simulink model "r2bb2xpfb14mcr25"  (R2012b)
settings: Solver=VariableStepDiscrete  SolverMode=SingleTasking  StartTime=0.0  StopTime=10.0  RelTol=1e-3
undefined symbols (not defined in the file): bit_reverse, pfb_coeff_gen_calc
libraries: xbsIndex_r4 x8058, casper_library_misc x54, casper_library_delays x18, xps_library x7
(part 92 of 105)

== system r2bb2xpfb14mcr25/fft_biplex_2by2_real/fft_biplex_real_2x2/biplex_core/fft_stage_14/butterfly_direct/twiddle/coeff_gen/cosin ==
  theta : Inport
  misci : Inport  Port=2
  Constant4 : xbsIndex_r4/Constant  const=0  gui_display_data_type=Fixed-point  arith_type=Unsigned  n_bits=1  bin_pt=0  preci_type=Single  exp_width=8  frac_width=24  explicit_period=on  period=1  equ=P=C  opselect=C  inp2=PCIN>>17  opr=+  inp1=P  carry=CIN  dbl_ovrd=off  block_type=constant
  Constant5 : xbsIndex_r4/Constant  const=0  gui_display_data_type=Fixed-point  arith_type=Unsigned  n_bits=1  bin_pt=0  preci_type=Single  exp_width=8  frac_width=24  explicit_period=on  period=1  equ=P=C  opselect=C  inp2=PCIN>>17  opr=+  inp1=P  carry=CIN  dbl_ovrd=off  block_type=constant
  Delay : xbsIndex_r4/Delay  rst=off  infoeditControl=Selection of Reset will increase slice count due to use of real FFs and instead of SRLs  en=off  latency=bram_latency  dbl_ovrd=off  reg_retiming=on  block_type=delay
  Delay10 : xbsIndex_r4/Delay  rst=off  infoeditControl=Selection of Reset will increase slice count due to use of real FFs and instead of SRLs  en=off  latency=bram_latency  dbl_ovrd=off  reg_retiming=on  block_type=delay
  Delay8 : xbsIndex_r4/Delay  rst=off  infoeditControl=Selection of Reset will increase slice count due to use of real FFs and instead of SRLs  en=off  latency=bram_latency  dbl_ovrd=off  reg_retiming=on  block_type=delay
  ROM : xbsIndex_r4/ROM  depth=2^(13)  initVector=[34359476224 34359738318 34359738267 34359738217 34359738167 34359738117 34359738066 34359738016 34359737966 34359737916 34359737865 34359737815 34359737765 34359475571 34359475520 34359475470 34359475420 34359213225 34359213175 34359213125 34358950931 34358950880 34358688686 34358688636 34358426442 34358426391 34358164197 34358164147 34357901953 34357901902 34357639708 34357639658 34357377464 34357377413 34357115219 34356853025 34356852975 34356590780 34356328586 34356066392 34356066341 34355804147 34355541953 34355279759 34355017564 34354755370 34354755320 34354493126 34354230931 34353968737 34353706543 34353444349 34353182154 34352919960 34352657766 34352395572 34352133377 34351871183 34351608989 34351084651 34350822456 34350560262 34350298068 34350035874 34349773679 34349249341 34348987147 34348724953 34348200614 34347938420 34347676226 34347151888 34346889693 34346627499 34346103161 34345840967 34345316628 34345054434 34344530096 34344267902 34343743563 34343481369 34342957031 34342694837 34342170498 34341646160 34341383966 34340859628 34340335289 34340073095 34339548757 34339024419 34338500081 34338237886 34337713548 34337189210 34336664872 34336140533 34335616195 34335354001 34334829663 34334305324 34333780986 34333256648 34332732310 34332207972 34331683633 34331159295 34330634957 34330110619 34329324136 34328799798 34328275460 34327751122 34327226784 34326702445 34325915963 34325391625 34324867287 34324342948 34323556466 34323032128 34322507790 34321721308 34321196969 34320410487 34319886149 34319361811 34318575329 34318050990 34317264508 34316740170 34315953688 34315429350 34314642867 34313856385 34313332047 34312545565 34311759083 34311234744 34310448262 34309661780 34309137442 34308350960 34307564477 34306777995 34306253657 34305467175 34304680693 34303894211 34303107728 34302321246 34301534764 34300748282 34299961800 34299437461 34298650979 34297602353 34296815871 34296029389 34295242907 34294456424 34293669942 34292883460 34292096978 34291310496 34290261870 34289475387 34288688905 34287902423 34287115941 34286067315 34285280833 34284494350 34283445724 34282659242 34281872760 34280824134 34280037652 34278989026 34278202543 34277153917 34276367435 34275318809 34274532327 34273483701 34272697219 34271648592 34270599966 34269813484 34268764858 34267978376 34266929750 34265881124 34264832497 34264046015 34262997389 34261948763 34260900137 34259851511 34259065029 34258016403 34256967777 34255919150 34254870524 34253821898 34252773272 34251724646 34250676020 34249627394 34248578768 34247530142 34246481515 34245432889 34244384263 34243335637 34242287011 34240976241 34239927615 34238878989 34237830363 34236781737 34235470967 34234422340 34233373714 34232062944 34231014318 34229965692 34228654922 34227606296 34226295526 34225246900 34224198274 34222887504 34221838878 34220528108 34219479482 34218168711 34216857941 34215809315 34214498545 34213449919 34212139149 34210828379 34209779753 34208468983 34207158213 34205847443 34204798817 34203488047 34202177277 34200866507 34199555737 34198507111 34197196341 34195885571 34194574801 34193264031 34191953261 34190642491 34189331721 34188020951 34186710181 34185399411 34184088641 34182777871 34181467101 34179894187 34178583417 34177272647 34175961877 34174651107 34173340337 34171767423 34170456653 34169145883 34167572969 34166262199 34164951429 34163378515 34162067745 34160756975 34159184061 34157873291 34156300377 34154989607 34153416693 34152105923 34150533009 34149222239 34147649325 34146338555 34144765641 34143192727 34141881957 34140309043 34138736129 34137425359 34135852445 34134279532 34132968762 34131395848 34129822934 34128250020 34126677106 34125104192 34123793422 34122220508 34120647594 34119074680 34117501766 34115928852 34114355939 34112783025 34111210111 34109637197 34108064283 34106491369 34104918455 34103083397 34101510483 34099937570 34098364656 34096791742 34095218828 34093383770 34091810856 34090237942 34088402884 34086829970 34085257057 34083421999 34081849085 ...(+93451 chars)]  distributed_mem=Block RAM  rst=off  init_reg=0  en=off  latency=bram_latency  gui_display_data_type=Fixed-point  arith_type=Unsigned  n_bits=n_bits*2  bin_pt=0  preci_type=Single  exp_width=8  frac_width=24  dbl_ovrd=off  optimize=Speed  use_rpm=on  block_type=sprom
  Terminator : Terminator
  Terminator1 : Terminator
  Terminator4 : Terminator
  add_convert0 : Subsystem
  add_convert1 : Subsystem
  assert : xbsIndex_r4/Assert  assert_type=on  type_source=Explicitly  gui_display_data_type=Fixed-point  arith_type=Unsigned  n_bits=13  bin_pt=0  preci_type=Single  exp_width=8  frac_width=24  assert_rate=off  rate_source=Explicitly  period=1  output_port=on  block_type=assert
  c_to_ri : casper_library_misc/c_to_ri  n_bits=n_bits  bin_pt=bin_pt
  invert0 : Subsystem  mask{n_bits=n_bits, bin_pt=bin_pt, neg_latency=neg_latency, mux_latency=mux_latency}
      mask prompts: n_bits "bit width"; bin_pt "binary point"; neg_latency "negate latency"; mux_latency "mux latency"
  invert1 : Subsystem  mask{n_bits=n_bits, bin_pt=bin_pt, neg_latency=neg_latency, mux_latency=mux_latency}
      mask prompts: n_bits "bit width"; bin_pt "binary point"; neg_latency "negate latency"; mux_latency "mux latency"
  cos : Outport
  -sin : Outport  Port=2
  misco : Outport  Port=3
  wires:
  theta/1 -> assert/1
  assert/1 -> add_convert0/1(theta), add_convert1/1(theta)
  Constant4/1 -> add_convert0/2(misci)
  add_convert0/3(misco) -> Terminator/1
  misci/1 -> add_convert1/2(misci)
  add_convert1/3(misco) -> Delay/1
  add_convert0/2(add) -> ROM/1
  add_convert1/2(add) -> Terminator4/1
  ROM/1 -> c_to_ri/1
  add_convert1/1(negate) -> Delay8/1
  add_convert0/1(negate) -> Delay10/1
  Delay10/1 -> invert0/1(negate)
  Constant5/1 -> invert0/3(misci)
  c_to_ri/1 -> invert0/2(in)
  Delay8/1 -> invert1/1(negate)
  c_to_ri/2 -> invert1/2(in)
  invert0/2(misco) -> Terminator1/1
  Delay/1 -> invert1/3(misci)
  invert0/1(out) -> cos/1
  invert1/1(out) -> -sin/1
  invert1/2(misco) -> misco/1
